simulink model "HW7_2"  (R2021a)
settings: Solver=VariableStepAuto  StartTime=0.0  StopTime=80  RelTol=1e-3
undefined symbols (not defined in the file): f, f_64
libraries: hdlBasic x991, xbsIndex_r4 x1, simulink x1
(part 6 of 6)

== system HW7_2/FIR_64/FIR-transposed1 ==
  In1 : Inport
  In2 : Inport  Port=2
  AddSub{7..11} (5 alike) : hdlBasic/AddSub  mode=Addition  use_carryin=off  use_carryout=off  en=off  latency=0  precision=User Defined  arith_type="Signed  (2's comp)"  n_bits=16  bin_pt=8  quantization=Truncate  overflow=Saturate  use_behavioral_HDL=off  hw_selection=Fabric  pipelined=off  XmcBlockStatus=1  maskContainerNames=tabcontainer1  block_type=addsub  block_config=sysgen:Addsub_config
  AddSub12 : hdlBasic/AddSub  mode=Addition  use_carryin=off  use_carryout=off  en=off  latency=0  precision=User Defined  arith_type=Unsigned  n_bits=16  bin_pt=8  quantization=Truncate  overflow=Saturate  use_behavioral_HDL=off  hw_selection=Fabric  pipelined=off  XmcBlockStatus=1  maskContainerNames=tabcontainer1  block_type=addsub  block_config=sysgen:Addsub_config
  CMult10 : hdlBasic/CMult  const=f(5)  gui_display_data_type=Fixed-point  const_n_bits=8  const_bin_pt=4  float_type=Single  exp_bits=8  fraction_bits=24  en=off  latency=0  precision=User Defined  arith_type="Signed  (2's comp)"  n_bits=16  bin_pt=8  quantization=Truncate  overflow=Saturate  use_behavioral_HDL=off  mem_type=Block RAM  pipeline=off  XmcBlockStatus=1  maskContainerNames=tabcontainer1  block_type=cmult  block_config=sysgen:CMult_config
      settings: infoedit=[]
  CMult11 : hdlBasic/CMult  const=f(6)  gui_display_data_type=Fixed-point  const_n_bits=8  const_bin_pt=4  float_type=Single  exp_bits=8  fraction_bits=24  en=off  latency=0  precision=User Defined  arith_type="Signed  (2's comp)"  n_bits=16  bin_pt=8  quantization=Truncate  overflow=Saturate  use_behavioral_HDL=off  mem_type=Block RAM  pipeline=off  XmcBlockStatus=1  maskContainerNames=tabcontainer1  block_type=cmult  block_config=sysgen:CMult_config
      settings: infoedit=[]
  CMult12 : hdlBasic/CMult  const=f(4)  gui_display_data_type=Fixed-point  const_n_bits=8  const_bin_pt=4  float_type=Single  exp_bits=8  fraction_bits=24  en=off  latency=0  precision=User Defined  arith_type="Signed  (2's comp)"  n_bits=16  bin_pt=8  quantization=Truncate  overflow=Saturate  use_behavioral_HDL=off  mem_type=Block RAM  pipeline=off  XmcBlockStatus=1  maskContainerNames=tabcontainer1  block_type=cmult  block_config=sysgen:CMult_config
      settings: infoedit=[]
  CMult13 : hdlBasic/CMult  const=f(3)  gui_display_data_type=Fixed-point  const_n_bits=8  const_bin_pt=4  float_type=Single  exp_bits=8  fraction_bits=24  en=off  latency=0  precision=User Defined  arith_type="Signed  (2's comp)"  n_bits=16  bin_pt=8  quantization=Truncate  overflow=Saturate  use_behavioral_HDL=off  mem_type=Block RAM  pipeline=off  XmcBlockStatus=1  maskContainerNames=tabcontainer1  block_type=cmult  block_config=sysgen:CMult_config
      settings: infoedit=[]
  CMult14 : hdlBasic/CMult  const=f(2)  gui_display_data_type=Fixed-point  const_n_bits=8  const_bin_pt=4  float_type=Single  exp_bits=8  fraction_bits=24  en=off  latency=0  precision=User Defined  arith_type="Signed  (2's comp)"  n_bits=16  bin_pt=8  quantization=Truncate  overflow=Saturate  use_behavioral_HDL=off  mem_type=Block RAM  pipeline=off  XmcBlockStatus=1  maskContainerNames=tabcontainer1  block_type=cmult  block_config=sysgen:CMult_config
      settings: infoedit=[]
  CMult15 : hdlBasic/CMult  const=f(1)  gui_display_data_type=Fixed-point  const_n_bits=8  const_bin_pt=4  float_type=Single  exp_bits=8  fraction_bits=24  en=off  latency=0  precision=User Defined  arith_type="Signed  (2's comp)"  n_bits=16  bin_pt=8  quantization=Truncate  overflow=Saturate  use_behavioral_HDL=off  mem_type=Block RAM  pipeline=off  XmcBlockStatus=1  maskContainerNames=tabcontainer1  block_type=cmult  block_config=sysgen:CMult_config
      settings: infoedit=[]
  CMult8 : hdlBasic/CMult  const=f(8)  gui_display_data_type=Fixed-point  const_n_bits=8  const_bin_pt=4  float_type=Single  exp_bits=8  fraction_bits=24  en=off  latency=0  precision=User Defined  arith_type="Signed  (2's comp)"  n_bits=16  bin_pt=8  quantization=Truncate  overflow=Saturate  use_behavioral_HDL=off  mem_type=Block RAM  pipeline=off  XmcBlockStatus=1  maskContainerNames=tabcontainer1  block_type=cmult  block_config=sysgen:CMult_config
      settings: infoedit=[]
  CMult9 : hdlBasic/CMult  const=f(7)  gui_display_data_type=Fixed-point  const_n_bits=8  const_bin_pt=4  float_type=Single  exp_bits=8  fraction_bits=24  en=off  latency=0  precision=User Defined  arith_type="Signed  (2's comp)"  n_bits=16  bin_pt=8  quantization=Truncate  overflow=Saturate  use_behavioral_HDL=off  mem_type=Block RAM  pipeline=off  XmcBlockStatus=1  maskContainerNames=tabcontainer1  block_type=cmult  block_config=sysgen:CMult_config
      settings: infoedit=[]
  Delay{1,7..13} (8 alike) : hdlBasic/Delay  rst=off  en=off  latency=1  reg_retiming=off  XmcBlockStatus=1  maskContainerNames=group1  block_type=delay  block_config=sysgen:Delay_config
  Transposed : hdlBasic/AddSub  mode=Addition  use_carryin=off  use_carryout=off  en=off  latency=0  precision=User Defined  arith_type="Signed  (2's comp)"  n_bits=16  bin_pt=8  quantization=Truncate  overflow=Saturate  use_behavioral_HDL=off  hw_selection=Fabric  pipelined=off  XmcBlockStatus=1  maskContainerNames=tabcontainer1  block_type=addsub  block_config=sysgen:Addsub_config
  Transposed1 : hdlBasic/AddSub  mode=Addition  use_carryin=off  use_carryout=off  en=off  latency=0  precision=User Defined  arith_type="Signed  (2's comp)"  n_bits=16  bin_pt=8  quantization=Truncate  overflow=Saturate  use_behavioral_HDL=off  hw_selection=Fabric  pipelined=off  XmcBlockStatus=1  maskContainerNames=tabcontainer1  block_type=addsub  block_config=sysgen:Addsub_config
  Out1 : Outport
  Out2 : Outport  Port=2
  wires:
  Delay12/1 -> AddSub12/2
  CMult10/1 -> AddSub9/1
  AddSub12/1 -> Delay13/1
  Delay9/1 -> AddSub9/2
  CMult9/1 -> AddSub7/1
  AddSub11/1 -> Delay12/1
  Delay10/1 -> AddSub10/2
  AddSub8/1 -> Delay9/1
  CMult11/1 -> AddSub8/1
  Delay8/1 -> AddSub8/2
  CMult12/1 -> AddSub10/1
  Delay11/1 -> AddSub11/2
  AddSub10/1 -> Delay11/1
  CMult14/1 -> AddSub12/1
  CMult15/1 -> Transposed/1
  Delay7/1 -> AddSub7/2
  CMult13/1 -> AddSub11/1
  Delay13/1 -> Transposed/2
  AddSub7/1 -> Delay8/1
  AddSub9/1 -> Delay10/1
  In1/1 -> CMult8/1, Out1/1, CMult15/1, CMult14/1, CMult13/1, CMult12/1, CMult10/1, CMult11/1, CMult9/1
  Transposed/1 -> Out2/1
  Transposed1/1 -> Delay7/1
  CMult8/1 -> Transposed1/1
  Delay1/1 -> Transposed1/2
  In2/1 -> Delay1/1

== system HW7_2/FIR_64/FIR-transposed2 ==
  In1 : Inport
  In2 : Inport  Port=2
  AddSub{7..11} (5 alike) : hdlBasic/AddSub  mode=Addition  use_carryin=off  use_carryout=off  en=off  latency=0  precision=User Defined  arith_type="Signed  (2's comp)"  n_bits=16  bin_pt=8  quantization=Truncate  overflow=Saturate  use_behavioral_HDL=off  hw_selection=Fabric  pipelined=off  XmcBlockStatus=1  maskContainerNames=tabcontainer1  block_type=addsub  block_config=sysgen:Addsub_config
  AddSub12 : hdlBasic/AddSub  mode=Addition  use_carryin=off  use_carryout=off  en=off  latency=0  precision=User Defined  arith_type=Unsigned  n_bits=16  bin_pt=8  quantization=Truncate  overflow=Saturate  use_behavioral_HDL=off  hw_selection=Fabric  pipelined=off  XmcBlockStatus=1  maskContainerNames=tabcontainer1  block_type=addsub  block_config=sysgen:Addsub_config
  CMult10 : hdlBasic/CMult  const=f(5)  gui_display_data_type=Fixed-point  const_n_bits=8  const_bin_pt=4  float_type=Single  exp_bits=8  fraction_bits=24  en=off  latency=0  precision=User Defined  arith_type="Signed  (2's comp)"  n_bits=16  bin_pt=8  quantization=Truncate  overflow=Saturate  use_behavioral_HDL=off  mem_type=Block RAM  pipeline=off  XmcBlockStatus=1  maskContainerNames=tabcontainer1  block_type=cmult  block_config=sysgen:CMult_config
      settings: infoedit=[]
  CMult11 : hdlBasic/CMult  const=f(6)  gui_display_data_type=Fixed-point  const_n_bits=8  const_bin_pt=4  float_type=Single  exp_bits=8  fraction_bits=24  en=off  latency=0  precision=User Defined  arith_type="Signed  (2's comp)"  n_bits=16  bin_pt=8  quantization=Truncate  overflow=Saturate  use_behavioral_HDL=off  mem_type=Block RAM  pipeline=off  XmcBlockStatus=1  maskContainerNames=tabcontainer1  block_type=cmult  block_config=sysgen:CMult_config
      settings: infoedit=[]
  CMult12 : hdlBasic/CMult  const=f(4)  gui_display_data_type=Fixed-point  const_n_bits=8  const_bin_pt=4  float_type=Single  exp_bits=8  fraction_bits=24  en=off  latency=0  precision=User Defined  arith_type="Signed  (2's comp)"  n_bits=16  bin_pt=8  quantization=Truncate  overflow=Saturate  use_behavioral_HDL=off  mem_type=Block RAM  pipeline=off  XmcBlockStatus=1  maskContainerNames=tabcontainer1  block_type=cmult  block_config=sysgen:CMult_config
      settings: infoedit=[]
  CMult13 : hdlBasic/CMult  const=f(3)  gui_display_data_type=Fixed-point  const_n_bits=8  const_bin_pt=4  float_type=Single  exp_bits=8  fraction_bits=24  en=off  latency=0  precision=User Defined  arith_type="Signed  (2's comp)"  n_bits=16  bin_pt=8  quantization=Truncate  overflow=Saturate  use_behavioral_HDL=off  mem_type=Block RAM  pipeline=off  XmcBlockStatus=1  maskContainerNames=tabcontainer1  block_type=cmult  block_config=sysgen:CMult_config
      settings: infoedit=[]
  CMult14 : hdlBasic/CMult  const=f(2)  gui_display_data_type=Fixed-point  const_n_bits=8  const_bin_pt=4  float_type=Single  exp_bits=8  fraction_bits=24  en=off  latency=0  precision=User Defined  arith_type="Signed  (2's comp)"  n_bits=16  bin_pt=8  quantization=Truncate  overflow=Saturate  use_behavioral_HDL=off  mem_type=Block RAM  pipeline=off  XmcBlockStatus=1  maskContainerNames=tabcontainer1  block_type=cmult  block_config=sysgen:CMult_config
      settings: infoedit=[]
  CMult15 : hdlBasic/CMult  const=f(1)  gui_display_data_type=Fixed-point  const_n_bits=8  const_bin_pt=4  float_type=Single  exp_bits=8  fraction_bits=24  en=off  latency=0  precision=User Defined  arith_type="Signed  (2's comp)"  n_bits=16  bin_pt=8  quantization=Truncate  overflow=Saturate  use_behavioral_HDL=off  mem_type=Block RAM  pipeline=off  XmcBlockStatus=1  maskContainerNames=tabcontainer1  block_type=cmult  block_config=sysgen:CMult_config
      settings: infoedit=[]
  CMult8 : hdlBasic/CMult  const=f(8)  gui_display_data_type=Fixed-point  const_n_bits=8  const_bin_pt=4  float_type=Single  exp_bits=8  fraction_bits=24  en=off  latency=0  precision=User Defined  arith_type="Signed  (2's comp)"  n_bits=16  bin_pt=8  quantization=Truncate  overflow=Saturate  use_behavioral_HDL=off  mem_type=Block RAM  pipeline=off  XmcBlockStatus=1  maskContainerNames=tabcontainer1  block_type=cmult  block_config=sysgen:CMult_config
      settings: infoedit=[]
  CMult9 : hdlBasic/CMult  const=f(7)  gui_display_data_type=Fixed-point  const_n_bits=8  const_bin_pt=4  float_type=Single  exp_bits=8  fraction_bits=24  en=off  latency=0  precision=User Defined  arith_type="Signed  (2's comp)"  n_bits=16  bin_pt=8  quantization=Truncate  overflow=Saturate  use_behavioral_HDL=off  mem_type=Block RAM  pipeline=off  XmcBlockStatus=1  maskContainerNames=tabcontainer1  block_type=cmult  block_config=sysgen:CMult_config
      settings: infoedit=[]
  Delay{1,7..13} (8 alike) : hdlBasic/Delay  rst=off  en=off  latency=1  reg_retiming=off  XmcBlockStatus=1  maskContainerNames=group1  block_type=delay  block_config=sysgen:Delay_config
  Transposed : hdlBasic/AddSub  mode=Addition  use_carryin=off  use_carryout=off  en=off  latency=0  precision=User Defined  arith_type="Signed  (2's comp)"  n_bits=16  bin_pt=8  quantization=Truncate  overflow=Saturate  use_behavioral_HDL=off  hw_selection=Fabric  pipelined=off  XmcBlockStatus=1  maskContainerNames=tabcontainer1  block_type=addsub  block_config=sysgen:Addsub_config
  Transposed1 : hdlBasic/AddSub  mode=Addition  use_carryin=off  use_carryout=off  en=off  latency=0  precision=User Defined  arith_type="Signed  (2's comp)"  n_bits=16  bin_pt=8  quantization=Truncate  overflow=Saturate  use_behavioral_HDL=off  hw_selection=Fabric  pipelined=off  XmcBlockStatus=1  maskContainerNames=tabcontainer1  block_type=addsub  block_config=sysgen:Addsub_config
  Out1 : Outport
  Out2 : Outport  Port=2
  wires:
  Delay12/1 -> AddSub12/2
  CMult10/1 -> AddSub9/1
  AddSub12/1 -> Delay13/1
  Delay9/1 -> AddSub9/2
  CMult9/1 -> AddSub7/1
  AddSub11/1 -> Delay12/1
  Delay10/1 -> AddSub10/2
  AddSub8/1 -> Delay9/1
  CMult11/1 -> AddSub8/1
  Delay8/1 -> AddSub8/2
  CMult12/1 -> AddSub10/1
  Delay11/1 -> AddSub11/2
  AddSub10/1 -> Delay11/1
  CMult14/1 -> AddSub12/1
  CMult15/1 -> Transposed/1
  Delay7/1 -> AddSub7/2
  CMult13/1 -> AddSub11/1
  Delay13/1 -> Transposed/2
  AddSub7/1 -> Delay8/1
  AddSub9/1 -> Delay10/1
  In1/1 -> CMult8/1, Out1/1, CMult15/1, CMult14/1, CMult13/1, CMult12/1, CMult10/1, CMult11/1, CMult9/1
  Transposed/1 -> Out2/1
  Transposed1/1 -> Delay7/1
  CMult8/1 -> Transposed1/1
  Delay1/1 -> Transposed1/2
  In2/1 -> Delay1/1

== system HW7_2/FIR_64/FIR-transposed3 ==
  In1 : Inport
  In2 : Inport  Port=2
  AddSub{7..11} (5 alike) : hdlBasic/AddSub  mode=Addition  use_carryin=off  use_carryout=off  en=off  latency=0  precision=User Defined  arith_type="Signed  (2's comp)"  n_bits=16  bin_pt=8  quantization=Truncate  overflow=Saturate  use_behavioral_HDL=off  hw_selection=Fabric  pipelined=off  XmcBlockStatus=1  maskContainerNames=tabcontainer1  block_type=addsub  block_config=sysgen:Addsub_config
  AddSub12 : hdlBasic/AddSub  mode=Addition  use_carryin=off  use_carryout=off  en=off  latency=0  precision=User Defined  arith_type=Unsigned  n_bits=16  bin_pt=8  quantization=Truncate  overflow=Saturate  use_behavioral_HDL=off  hw_selection=Fabric  pipelined=off  XmcBlockStatus=1  maskContainerNames=tabcontainer1  block_type=addsub  block_config=sysgen:Addsub_config
  CMult10 : hdlBasic/CMult  const=f(5)  gui_display_data_type=Fixed-point  const_n_bits=8  const_bin_pt=4  float_type=Single  exp_bits=8  fraction_bits=24  en=off  latency=0  precision=User Defined  arith_type="Signed  (2's comp)"  n_bits=16  bin_pt=8  quantization=Truncate  overflow=Saturate  use_behavioral_HDL=off  mem_type=Block RAM  pipeline=off  XmcBlockStatus=1  maskContainerNames=tabcontainer1  block_type=cmult  block_config=sysgen:CMult_config
      settings: infoedit=[]
  CMult11 : hdlBasic/CMult  const=f(6)  gui_display_data_type=Fixed-point  const_n_bits=8  const_bin_pt=4  float_type=Single  exp_bits=8  fraction_bits=24  en=off  latency=0  precision=User Defined  arith_type="Signed  (2's comp)"  n_bits=16  bin_pt=8  quantization=Truncate  overflow=Saturate  use_behavioral_HDL=off  mem_type=Block RAM  pipeline=off  XmcBlockStatus=1  maskContainerNames=tabcontainer1  block_type=cmult  block_config=sysgen:CMult_config
      settings: infoedit=[]
  CMult12 : hdlBasic/CMult  const=f(4)  gui_display_data_type=Fixed-point  const_n_bits=8  const_bin_pt=4  float_type=Single  exp_bits=8  fraction_bits=24  en=off  latency=0  precision=User Defined  arith_type="Signed  (2's comp)"  n_bits=16  bin_pt=8  quantization=Truncate  overflow=Saturate  use_behavioral_HDL=off  mem_type=Block RAM  pipeline=off  XmcBlockStatus=1  maskContainerNames=tabcontainer1  block_type=cmult  block_config=sysgen:CMult_config
      settings: infoedit=[]
  CMult13 : hdlBasic/CMult  const=f(3)  gui_display_data_type=Fixed-point  const_n_bits=8  const_bin_pt=4  float_type=Single  exp_bits=8  fraction_bits=24  en=off  latency=0  precision=User Defined  arith_type="Signed  (2's comp)"  n_bits=16  bin_pt=8  quantization=Truncate  overflow=Saturate  use_behavioral_HDL=off  mem_type=Block RAM  pipeline=off  XmcBlockStatus=1  maskContainerNames=tabcontainer1  block_type=cmult  block_config=sysgen:CMult_config
      settings: infoedit=[]
  CMult14 : hdlBasic/CMult  const=f(2)  gui_display_data_type=Fixed-point  const_n_bits=8  const_bin_pt=4  float_type=Single  exp_bits=8  fraction_bits=24  en=off  latency=0  precision=User Defined  arith_type="Signed  (2's comp)"  n_bits=16  bin_pt=8  quantization=Truncate  overflow=Saturate  use_behavioral_HDL=off  mem_type=Block RAM  pipeline=off  XmcBlockStatus=1  maskContainerNames=tabcontainer1  block_type=cmult  block_config=sysgen:CMult_config
      settings: infoedit=[]
  CMult15 : hdlBasic/CMult  const=f(1)  gui_display_data_type=Fixed-point  const_n_bits=8  const_bin_pt=4  float_type=Single  exp_bits=8  fraction_bits=24  en=off  latency=0  precision=User Defined  arith_type="Signed  (2's comp)"  n_bits=16  bin_pt=8  quantization=Truncate  overflow=Saturate  use_behavioral_HDL=off  mem_type=Block RAM  pipeline=off  XmcBlockStatus=1  maskContainerNames=tabcontainer1  block_type=cmult  block_config=sysgen:CMult_config
      settings: infoedit=[]
  CMult8 : hdlBasic/CMult  const=f(8)  gui_display_data_type=Fixed-point  const_n_bits=8  const_bin_pt=4  float_type=Single  exp_bits=8  fraction_bits=24  en=off  latency=0  precision=User Defined  arith_type="Signed  (2's comp)"  n_bits=16  bin_pt=8  quantization=Truncate  overflow=Saturate  use_behavioral_HDL=off  mem_type=Block RAM  pipeline=off  XmcBlockStatus=1  maskContainerNames=tabcontainer1  block_type=cmult  block_config=sysgen:CMult_config
      settings: infoedit=[]
  CMult9 : hdlBasic/CMult  const=f(7)  gui_display_data_type=Fixed-point  const_n_bits=8  const_bin_pt=4  float_type=Single  exp_bits=8  fraction_bits=24  en=off  latency=0  precision=User Defined  arith_type="Signed  (2's comp)"  n_bits=16  bin_pt=8  quantization=Truncate  overflow=Saturate  use_behavioral_HDL=off  mem_type=Block RAM  pipeline=off  XmcBlockStatus=1  maskContainerNames=tabcontainer1  block_type=cmult  block_config=sysgen:CMult_config
      settings: infoedit=[]
  Delay{1,7..13} (8 alike) : hdlBasic/Delay  rst=off  en=off  latency=1  reg_retiming=off  XmcBlockStatus=1  maskContainerNames=group1  block_type=delay  block_config=sysgen:Delay_config
  Transposed : hdlBasic/AddSub  mode=Addition  use_carryin=off  use_carryout=off  en=off  latency=0  precision=User Defined  arith_type="Signed  (2's comp)"  n_bits=16  bin_pt=8  quantization=Truncate  overflow=Saturate  use_behavioral_HDL=off  hw_selection=Fabric  pipelined=off  XmcBlockStatus=1  maskContainerNames=tabcontainer1  block_type=addsub  block_config=sysgen:Addsub_config
  Transposed1 : hdlBasic/AddSub  mode=Addition  use_carryin=off  use_carryout=off  en=off  latency=0  precision=User Defined  arith_type="Signed  (2's comp)"  n_bits=16  bin_pt=8  quantization=Truncate  overflow=Saturate  use_behavioral_HDL=off  hw_selection=Fabric  pipelined=off  XmcBlockStatus=1  maskContainerNames=tabcontainer1  block_type=addsub  block_config=sysgen:Addsub_config
  Out1 : Outport
  Out2 : Outport  Port=2
  wires:
  Delay12/1 -> AddSub12/2
  CMult10/1 -> AddSub9/1
  AddSub12/1 -> Delay13/1
  Delay9/1 -> AddSub9/2
  CMult9/1 -> AddSub7/1
  AddSub11/1 -> Delay12/1
  Delay10/1 -> AddSub10/2
  AddSub8/1 -> Delay9/1
  CMult11/1 -> AddSub8/1
  Delay8/1 -> AddSub8/2
  CMult12/1 -> AddSub10/1
  Delay11/1 -> AddSub11/2
  AddSub10/1 -> Delay11/1
  CMult14/1 -> AddSub12/1
  CMult15/1 -> Transposed/1
  Delay7/1 -> AddSub7/2
  CMult13/1 -> AddSub11/1
  Delay13/1 -> Transposed/2
  AddSub7/1 -> Delay8/1
  AddSub9/1 -> Delay10/1
  In1/1 -> CMult8/1, Out1/1, CMult15/1, CMult14/1, CMult13/1, CMult12/1, CMult10/1, CMult11/1, CMult9/1
  Transposed/1 -> Out2/1
  Transposed1/1 -> Delay7/1
  CMult8/1 -> Transposed1/1
  Delay1/1 -> Transposed1/2
  In2/1 -> Delay1/1

== system HW7_2/FIR_64/FIR-transposed4 ==
  In1 : Inport
  In2 : Inport  Port=2
  AddSub{7..11} (5 alike) : hdlBasic/AddSub  mode=Addition  use_carryin=off  use_carryout=off  en=off  latency=0  precision=User Defined  arith_type="Signed  (2's comp)"  n_bits=16  bin_pt=8  quantization=Truncate  overflow=Saturate  use_behavioral_HDL=off  hw_selection=Fabric  pipelined=off  XmcBlockStatus=1  maskContainerNames=tabcontainer1  block_type=addsub  block_config=sysgen:Addsub_config
  AddSub12 : hdlBasic/AddSub  mode=Addition  use_carryin=off  use_carryout=off  en=off  latency=0  precision=User Defined  arith_type=Unsigned  n_bits=16  bin_pt=8  quantization=Truncate  overflow=Saturate  use_behavioral_HDL=off  hw_selection=Fabric  pipelined=off  XmcBlockStatus=1  maskContainerNames=tabcontainer1  block_type=addsub  block_config=sysgen:Addsub_config
  CMult10 : hdlBasic/CMult  const=f(5)  gui_display_data_type=Fixed-point  const_n_bits=8  const_bin_pt=4  float_type=Single  exp_bits=8  fraction_bits=24  en=off  latency=0  precision=User Defined  arith_type="Signed  (2's comp)"  n_bits=16  bin_pt=8  quantization=Truncate  overflow=Saturate  use_behavioral_HDL=off  mem_type=Block RAM  pipeline=off  XmcBlockStatus=1  maskContainerNames=tabcontainer1  block_type=cmult  block_config=sysgen:CMult_config
      settings: infoedit=[]
  CMult11 : hdlBasic/CMult  const=f(6)  gui_display_data_type=Fixed-point  const_n_bits=8  const_bin_pt=4  float_type=Single  exp_bits=8  fraction_bits=24  en=off  latency=0  precision=User Defined  arith_type="Signed  (2's comp)"  n_bits=16  bin_pt=8  quantization=Truncate  overflow=Saturate  use_behavioral_HDL=off  mem_type=Block RAM  pipeline=off  XmcBlockStatus=1  maskContainerNames=tabcontainer1  block_type=cmult  block_config=sysgen:CMult_config
      settings: infoedit=[]
  CMult12 : hdlBasic/CMult  const=f(4)  gui_display_data_type=Fixed-point  const_n_bits=8  const_bin_pt=4  float_type=Single  exp_bits=8  fraction_bits=24  en=off  latency=0  precision=User Defined  arith_type="Signed  (2's comp)"  n_bits=16  bin_pt=8  quantization=Truncate  overflow=Saturate  use_behavioral_HDL=off  mem_type=Block RAM  pipeline=off  XmcBlockStatus=1  maskContainerNames=tabcontainer1  block_type=cmult  block_config=sysgen:CMult_config
      settings: infoedit=[]
  CMult13 : hdlBasic/CMult  const=f(3)  gui_display_data_type=Fixed-point  const_n_bits=8  const_bin_pt=4  float_type=Single  exp_bits=8  fraction_bits=24  en=off  latency=0  precision=User Defined  arith_type="Signed  (2's comp)"  n_bits=16  bin_pt=8  quantization=Truncate  overflow=Saturate  use_behavioral_HDL=off  mem_type=Block RAM  pipeline=off  XmcBlockStatus=1  maskContainerNames=tabcontainer1  block_type=cmult  block_config=sysgen:CMult_config
      settings: infoedit=[]
  CMult14 : hdlBasic/CMult  const=f(2)  gui_display_data_type=Fixed-point  const_n_bits=8  const_bin_pt=4  float_type=Single  exp_bits=8  fraction_bits=24  en=off  latency=0  precision=User Defined  arith_type="Signed  (2's comp)"  n_bits=16  bin_pt=8  quantization=Truncate  overflow=Saturate  use_behavioral_HDL=off  mem_type=Block RAM  pipeline=off  XmcBlockStatus=1  maskContainerNames=tabcontainer1  block_type=cmult  block_config=sysgen:CMult_config
      settings: infoedit=[]
  CMult15 : hdlBasic/CMult  const=f(1)  gui_display_data_type=Fixed-point  const_n_bits=8  const_bin_pt=4  float_type=Single  exp_bits=8  fraction_bits=24  en=off  latency=0  precision=User Defined  arith_type="Signed  (2's comp)"  n_bits=16  bin_pt=8  quantization=Truncate  overflow=Saturate  use_behavioral_HDL=off  mem_type=Block RAM  pipeline=off  XmcBlockStatus=1  maskContainerNames=tabcontainer1  block_type=cmult  block_config=sysgen:CMult_config
      settings: infoedit=[]
  CMult8 : hdlBasic/CMult  const=f(8)  gui_display_data_type=Fixed-point  const_n_bits=8  const_bin_pt=4  float_type=Single  exp_bits=8  fraction_bits=24  en=off  latency=0  precision=User Defined  arith_type="Signed  (2's comp)"  n_bits=16  bin_pt=8  quantization=Truncate  overflow=Saturate  use_behavioral_HDL=off  mem_type=Block RAM  pipeline=off  XmcBlockStatus=1  maskContainerNames=tabcontainer1  block_type=cmult  block_config=sysgen:CMult_config
      settings: infoedit=[]
  CMult9 : hdlBasic/CMult  const=f(7)  gui_display_data_type=Fixed-point  const_n_bits=8  const_bin_pt=4  float_type=Single  exp_bits=8  fraction_bits=24  en=off  latency=0  precision=User Defined  arith_type="Signed  (2's comp)"  n_bits=16  bin_pt=8  quantization=Truncate  overflow=Saturate  use_behavioral_HDL=off  mem_type=Block RAM  pipeline=off  XmcBlockStatus=1  maskContainerNames=tabcontainer1  block_type=cmult  block_config=sysgen:CMult_config
      settings: infoedit=[]
  Delay{1,7..13} (8 alike) : hdlBasic/Delay  rst=off  en=off  latency=1  reg_retiming=off  XmcBlockStatus=1  maskContainerNames=group1  block_type=delay  block_config=sysgen:Delay_config
  Transposed : hdlBasic/AddSub  mode=Addition  use_carryin=off  use_carryout=off  en=off  latency=0  precision=User Defined  arith_type="Signed  (2's comp)"  n_bits=16  bin_pt=8  quantization=Truncate  overflow=Saturate  use_behavioral_HDL=off  hw_selection=Fabric  pipelined=off  XmcBlockStatus=1  maskContainerNames=tabcontainer1  block_type=addsub  block_config=sysgen:Addsub_config
  Transposed1 : hdlBasic/AddSub  mode=Addition  use_carryin=off  use_carryout=off  en=off  latency=0  precision=User Defined  arith_type="Signed  (2's comp)"  n_bits=16  bin_pt=8  quantization=Truncate  overflow=Saturate  use_behavioral_HDL=off  hw_selection=Fabric  pipelined=off  XmcBlockStatus=1  maskContainerNames=tabcontainer1  block_type=addsub  block_config=sysgen:Addsub_config
  Out1 : Outport
  Out2 : Outport  Port=2
  wires:
  Delay12/1 -> AddSub12/2
  CMult10/1 -> AddSub9/1
  AddSub12/1 -> Delay13/1
  Delay9/1 -> AddSub9/2
  CMult9/1 -> AddSub7/1
  AddSub11/1 -> Delay12/1
  Delay10/1 -> AddSub10/2
  AddSub8/1 -> Delay9/1
  CMult11/1 -> AddSub8/1
  Delay8/1 -> AddSub8/2
  CMult12/1 -> AddSub10/1
  Delay11/1 -> AddSub11/2
  AddSub10/1 -> Delay11/1
  CMult14/1 -> AddSub12/1
  CMult15/1 -> Transposed/1
  Delay7/1 -> AddSub7/2
  CMult13/1 -> AddSub11/1
  Delay13/1 -> Transposed/2
  AddSub7/1 -> Delay8/1
  AddSub9/1 -> Delay10/1
  In1/1 -> CMult8/1, Out1/1, CMult15/1, CMult14/1, CMult13/1, CMult12/1, CMult10/1, CMult11/1, CMult9/1
  Transposed/1 -> Out2/1
  Transposed1/1 -> Delay7/1
  CMult8/1 -> Transposed1/1
  Delay1/1 -> Transposed1/2
  In2/1 -> Delay1/1

== system HW7_2/FIR_64/FIR-transposed5 ==
  In1 : Inport
  In2 : Inport  Port=2
  AddSub{7..11} (5 alike) : hdlBasic/AddSub  mode=Addition  use_carryin=off  use_carryout=off  en=off  latency=0  precision=User Defined  arith_type="Signed  (2's comp)"  n_bits=16  bin_pt=8  quantization=Truncate  overflow=Saturate  use_behavioral_HDL=off  hw_selection=Fabric  pipelined=off  XmcBlockStatus=1  maskContainerNames=tabcontainer1  block_type=addsub  block_config=sysgen:Addsub_config
  AddSub12 : hdlBasic/AddSub  mode=Addition  use_carryin=off  use_carryout=off  en=off  latency=0  precision=User Defined  arith_type=Unsigned  n_bits=16  bin_pt=8  quantization=Truncate  overflow=Saturate  use_behavioral_HDL=off  hw_selection=Fabric  pipelined=off  XmcBlockStatus=1  maskContainerNames=tabcontainer1  block_type=addsub  block_config=sysgen:Addsub_config
  CMult10 : hdlBasic/CMult  const=f(5)  gui_display_data_type=Fixed-point  const_n_bits=8  const_bin_pt=4  float_type=Single  exp_bits=8  fraction_bits=24  en=off  latency=0  precision=User Defined  arith_type="Signed  (2's comp)"  n_bits=16  bin_pt=8  quantization=Truncate  overflow=Saturate  use_behavioral_HDL=off  mem_type=Block RAM  pipeline=off  XmcBlockStatus=1  maskContainerNames=tabcontainer1  block_type=cmult  block_config=sysgen:CMult_config
      settings: infoedit=[]
  CMult11 : hdlBasic/CMult  const=f(6)  gui_display_data_type=Fixed-point  const_n_bits=8  const_bin_pt=4  float_type=Single  exp_bits=8  fraction_bits=24  en=off  latency=0  precision=User Defined  arith_type="Signed  (2's comp)"  n_bits=16  bin_pt=8  quantization=Truncate  overflow=Saturate  use_behavioral_HDL=off  mem_type=Block RAM  pipeline=off  XmcBlockStatus=1  maskContainerNames=tabcontainer1  block_type=cmult  block_config=sysgen:CMult_config
      settings: infoedit=[]
  CMult12 : hdlBasic/CMult  const=f(4)  gui_display_data_type=Fixed-point  const_n_bits=8  const_bin_pt=4  float_type=Single  exp_bits=8  fraction_bits=24  en=off  latency=0  precision=User Defined  arith_type="Signed  (2's comp)"  n_bits=16  bin_pt=8  quantization=Truncate  overflow=Saturate  use_behavioral_HDL=off  mem_type=Block RAM  pipeline=off  XmcBlockStatus=1  maskContainerNames=tabcontainer1  block_type=cmult  block_config=sysgen:CMult_config
      settings: infoedit=[]
  CMult13 : hdlBasic/CMult  const=f(3)  gui_display_data_type=Fixed-point  const_n_bits=8  const_bin_pt=4  float_type=Single  exp_bits=8  fraction_bits=24  en=off  latency=0  precision=User Defined  arith_type="Signed  (2's comp)"  n_bits=16  bin_pt=8  quantization=Truncate  overflow=Saturate  use_behavioral_HDL=off  mem_type=Block RAM  pipeline=off  XmcBlockStatus=1  maskContainerNames=tabcontainer1  block_type=cmult  block_config=sysgen:CMult_config
      settings: infoedit=[]
  CMult14 : hdlBasic/CMult  const=f(2)  gui_display_data_type=Fixed-point  const_n_bits=8  const_bin_pt=4  float_type=Single  exp_bits=8  fraction_bits=24  en=off  latency=0  precision=User Defined  arith_type="Signed  (2's comp)"  n_bits=16  bin_pt=8  quantization=Truncate  overflow=Saturate  use_behavioral_HDL=off  mem_type=Block RAM  pipeline=off  XmcBlockStatus=1  maskContainerNames=tabcontainer1  block_type=cmult  block_config=sysgen:CMult_config
      settings: infoedit=[]
  CMult15 : hdlBasic/CMult  const=f(1)  gui_display_data_type=Fixed-point  const_n_bits=8  const_bin_pt=4  float_type=Single  exp_bits=8  fraction_bits=24  en=off  latency=0  precision=User Defined  arith_type="Signed  (2's comp)"  n_bits=16  bin_pt=8  quantization=Truncate  overflow=Saturate  use_behavioral_HDL=off  mem_type=Block RAM  pipeline=off  XmcBlockStatus=1  maskContainerNames=tabcontainer1  block_type=cmult  block_config=sysgen:CMult_config
      settings: infoedit=[]
  CMult8 : hdlBasic/CMult  const=f(8)  gui_display_data_type=Fixed-point  const_n_bits=8  const_bin_pt=4  float_type=Single  exp_bits=8  fraction_bits=24  en=off  latency=0  precision=User Defined  arith_type="Signed  (2's comp)"  n_bits=16  bin_pt=8  quantization=Truncate  overflow=Saturate  use_behavioral_HDL=off  mem_type=Block RAM  pipeline=off  XmcBlockStatus=1  maskContainerNames=tabcontainer1  block_type=cmult  block_config=sysgen:CMult_config
      settings: infoedit=[]
  CMult9 : hdlBasic/CMult  const=f(7)  gui_display_data_type=Fixed-point  const_n_bits=8  const_bin_pt=4  float_type=Single  exp_bits=8  fraction_bits=24  en=off  latency=0  precision=User Defined  arith_type="Signed  (2's comp)"  n_bits=16  bin_pt=8  quantization=Truncate  overflow=Saturate  use_behavioral_HDL=off  mem_type=Block RAM  pipeline=off  XmcBlockStatus=1  maskContainerNames=tabcontainer1  block_type=cmult  block_config=sysgen:CMult_config
      settings: infoedit=[]
  Delay{1,7..13} (8 alike) : hdlBasic/Delay  rst=off  en=off  latency=1  reg_retiming=off  XmcBlockStatus=1  maskContainerNames=group1  block_type=delay  block_config=sysgen:Delay_config
  Transposed : hdlBasic/AddSub  mode=Addition  use_carryin=off  use_carryout=off  en=off  latency=0  precision=User Defined  arith_type="Signed  (2's comp)"  n_bits=16  bin_pt=8  quantization=Truncate  overflow=Saturate  use_behavioral_HDL=off  hw_selection=Fabric  pipelined=off  XmcBlockStatus=1  maskContainerNames=tabcontainer1  block_type=addsub  block_config=sysgen:Addsub_config
  Transposed1 : hdlBasic/AddSub  mode=Addition  use_carryin=off  use_carryout=off  en=off  latency=0  precision=User Defined  arith_type="Signed  (2's comp)"  n_bits=16  bin_pt=8  quantization=Truncate  overflow=Saturate  use_behavioral_HDL=off  hw_selection=Fabric  pipelined=off  XmcBlockStatus=1  maskContainerNames=tabcontainer1  block_type=addsub  block_config=sysgen:Addsub_config
  Out1 : Outport
  Out2 : Outport  Port=2
  wires:
  Delay12/1 -> AddSub12/2
  CMult10/1 -> AddSub9/1
  AddSub12/1 -> Delay13/1
  Delay9/1 -> AddSub9/2
  CMult9/1 -> AddSub7/1
  AddSub11/1 -> Delay12/1
  Delay10/1 -> AddSub10/2
  AddSub8/1 -> Delay9/1
  CMult11/1 -> AddSub8/1
  Delay8/1 -> AddSub8/2
  CMult12/1 -> AddSub10/1
  Delay11/1 -> AddSub11/2
  AddSub10/1 -> Delay11/1
  CMult14/1 -> AddSub12/1
  CMult15/1 -> Transposed/1
  Delay7/1 -> AddSub7/2
  CMult13/1 -> AddSub11/1
  Delay13/1 -> Transposed/2
  AddSub7/1 -> Delay8/1
  AddSub9/1 -> Delay10/1
  In1/1 -> CMult8/1, Out1/1, CMult15/1, CMult14/1, CMult13/1, CMult12/1, CMult10/1, CMult11/1, CMult9/1
  Transposed/1 -> Out2/1
  Transposed1/1 -> Delay7/1
  CMult8/1 -> Transposed1/1
  Delay1/1 -> Transposed1/2
  In2/1 -> Delay1/1

== system HW7_2/FIR_64/FIR-transposed6 ==
  In1 : Inport
  In2 : Inport  Port=2
  AddSub{7..11} (5 alike) : hdlBasic/AddSub  mode=Addition  use_carryin=off  use_carryout=off  en=off  latency=0  precision=User Defined  arith_type="Signed  (2's comp)"  n_bits=16  bin_pt=8  quantization=Truncate  overflow=Saturate  use_behavioral_HDL=off  hw_selection=Fabric  pipelined=off  XmcBlockStatus=1  maskContainerNames=tabcontainer1  block_type=addsub  block_config=sysgen:Addsub_config
  AddSub12 : hdlBasic/AddSub  mode=Addition  use_carryin=off  use_carryout=off  en=off  latency=0  precision=User Defined  arith_type=Unsigned  n_bits=16  bin_pt=8  quantization=Truncate  overflow=Saturate  use_behavioral_HDL=off  hw_selection=Fabric  pipelined=off  XmcBlockStatus=1  maskContainerNames=tabcontainer1  block_type=addsub  block_config=sysgen:Addsub_config
  CMult10 : hdlBasic/CMult  const=f(5)  gui_display_data_type=Fixed-point  const_n_bits=8  const_bin_pt=4  float_type=Single  exp_bits=8  fraction_bits=24  en=off  latency=0  precision=User Defined  arith_type="Signed  (2's comp)"  n_bits=16  bin_pt=8  quantization=Truncate  overflow=Saturate  use_behavioral_HDL=off  mem_type=Block RAM  pipeline=off  XmcBlockStatus=1  maskContainerNames=tabcontainer1  block_type=cmult  block_config=sysgen:CMult_config
      settings: infoedit=[]
  CMult11 : hdlBasic/CMult  const=f(6)  gui_display_data_type=Fixed-point  const_n_bits=8  const_bin_pt=4  float_type=Single  exp_bits=8  fraction_bits=24  en=off  latency=0  precision=User Defined  arith_type="Signed  (2's comp)"  n_bits=16  bin_pt=8  quantization=Truncate  overflow=Saturate  use_behavioral_HDL=off  mem_type=Block RAM  pipeline=off  XmcBlockStatus=1  maskContainerNames=tabcontainer1  block_type=cmult  block_config=sysgen:CMult_config
      settings: infoedit=[]
  CMult12 : hdlBasic/CMult  const=f(4)  gui_display_data_type=Fixed-point  const_n_bits=8  const_bin_pt=4  float_type=Single  exp_bits=8  fraction_bits=24  en=off  latency=0  precision=User Defined  arith_type="Signed  (2's comp)"  n_bits=16  bin_pt=8  quantization=Truncate  overflow=Saturate  use_behavioral_HDL=off  mem_type=Block RAM  pipeline=off  XmcBlockStatus=1  maskContainerNames=tabcontainer1  block_type=cmult  block_config=sysgen:CMult_config
      settings: infoedit=[]
  CMult13 : hdlBasic/CMult  const=f(3)  gui_display_data_type=Fixed-point  const_n_bits=8  const_bin_pt=4  float_type=Single  exp_bits=8  fraction_bits=24  en=off  latency=0  precision=User Defined  arith_type="Signed  (2's comp)"  n_bits=16  bin_pt=8  quantization=Truncate  overflow=Saturate  use_behavioral_HDL=off  mem_type=Block RAM  pipeline=off  XmcBlockStatus=1  maskContainerNames=tabcontainer1  block_type=cmult  block_config=sysgen:CMult_config
      settings: infoedit=[]
  CMult14 : hdlBasic/CMult  const=f(2)  gui_display_data_type=Fixed-point  const_n_bits=8  const_bin_pt=4  float_type=Single  exp_bits=8  fraction_bits=24  en=off  latency=0  precision=User Defined  arith_type="Signed  (2's comp)"  n_bits=16  bin_pt=8  quantization=Truncate  overflow=Saturate  use_behavioral_HDL=off  mem_type=Block RAM  pipeline=off  XmcBlockStatus=1  maskContainerNames=tabcontainer1  block_type=cmult  block_config=sysgen:CMult_config
      settings: infoedit=[]
  CMult15 : hdlBasic/CMult  const=f(1)  gui_display_data_type=Fixed-point  const_n_bits=8  const_bin_pt=4  float_type=Single  exp_bits=8  fraction_bits=24  en=off  latency=0  precision=User Defined  arith_type="Signed  (2's comp)"  n_bits=16  bin_pt=8  quantization=Truncate  overflow=Saturate  use_behavioral_HDL=off  mem_type=Block RAM  pipeline=off  XmcBlockStatus=1  maskContainerNames=tabcontainer1  block_type=cmult  block_config=sysgen:CMult_config
      settings: infoedit=[]
  CMult8 : hdlBasic/CMult  const=f(8)  gui_display_data_type=Fixed-point  const_n_bits=8  const_bin_pt=4  float_type=Single  exp_bits=8  fraction_bits=24  en=off  latency=0  precision=User Defined  arith_type="Signed  (2's comp)"  n_bits=16  bin_pt=8  quantization=Truncate  overflow=Saturate  use_behavioral_HDL=off  mem_type=Block RAM  pipeline=off  XmcBlockStatus=1  maskContainerNames=tabcontainer1  block_type=cmult  block_config=sysgen:CMult_config
      settings: infoedit=[]
  CMult9 : hdlBasic/CMult  const=f(7)  gui_display_data_type=Fixed-point  const_n_bits=8  const_bin_pt=4  float_type=Single  exp_bits=8  fraction_bits=24  en=off  latency=0  precision=User Defined  arith_type="Signed  (2's comp)"  n_bits=16  bin_pt=8  quantization=Truncate  overflow=Saturate  use_behavioral_HDL=off  mem_type=Block RAM  pipeline=off  XmcBlockStatus=1  maskContainerNames=tabcontainer1  block_type=cmult  block_config=sysgen:CMult_config
      settings: infoedit=[]
  Delay{1,7..13} (8 alike) : hdlBasic/Delay  rst=off  en=off  latency=1  reg_retiming=off  XmcBlockStatus=1  maskContainerNames=group1  block_type=delay  block_config=sysgen:Delay_config
  Transposed : hdlBasic/AddSub  mode=Addition  use_carryin=off  use_carryout=off  en=off  latency=0  precision=User Defined  arith_type="Signed  (2's comp)"  n_bits=16  bin_pt=8  quantization=Truncate  overflow=Saturate  use_behavioral_HDL=off  hw_selection=Fabric  pipelined=off  XmcBlockStatus=1  maskContainerNames=tabcontainer1  block_type=addsub  block_config=sysgen:Addsub_config
  Transposed1 : hdlBasic/AddSub  mode=Addition  use_carryin=off  use_carryout=off  en=off  latency=0  precision=User Defined  arith_type="Signed  (2's comp)"  n_bits=16  bin_pt=8  quantization=Truncate  overflow=Saturate  use_behavioral_HDL=off  hw_selection=Fabric  pipelined=off  XmcBlockStatus=1  maskContainerNames=tabcontainer1  block_type=addsub  block_config=sysgen:Addsub_config
  Out1 : Outport
  Out2 : Outport  Port=2
  wires:
  Delay12/1 -> AddSub12/2
  CMult10/1 -> AddSub9/1
  AddSub12/1 -> Delay13/1
  Delay9/1 -> AddSub9/2
  CMult9/1 -> AddSub7/1
  AddSub11/1 -> Delay12/1
  Delay10/1 -> AddSub10/2
  AddSub8/1 -> Delay9/1
  CMult11/1 -> AddSub8/1
  Delay8/1 -> AddSub8/2
  CMult12/1 -> AddSub10/1
  Delay11/1 -> AddSub11/2
  AddSub10/1 -> Delay11/1
  CMult14/1 -> AddSub12/1
  CMult15/1 -> Transposed/1
  Delay7/1 -> AddSub7/2
  CMult13/1 -> AddSub11/1
  Delay13/1 -> Transposed/2
  AddSub7/1 -> Delay8/1
  AddSub9/1 -> Delay10/1
  In1/1 -> CMult8/1, Out1/1, CMult15/1, CMult14/1, CMult13/1, CMult12/1, CMult10/1, CMult11/1, CMult9/1
  Transposed/1 -> Out2/1
  Transposed1/1 -> Delay7/1
  CMult8/1 -> Transposed1/1
  Delay1/1 -> Transposed1/2
  In2/1 -> Delay1/1

== system HW7_2/FIR_64/FIR-transposed7 ==
  In1 : Inport
  In2 : Inport  Port=2
  AddSub{7..11} (5 alike) : hdlBasic/AddSub  mode=Addition  use_carryin=off  use_carryout=off  en=off  latency=0  precision=User Defined  arith_type="Signed  (2's comp)"  n_bits=16  bin_pt=8  quantization=Truncate  overflow=Saturate  use_behavioral_HDL=off  hw_selection=Fabric  pipelined=off  XmcBlockStatus=1  maskContainerNames=tabcontainer1  block_type=addsub  block_config=sysgen:Addsub_config
  AddSub12 : hdlBasic/AddSub  mode=Addition  use_carryin=off  use_carryout=off  en=off  latency=0  precision=User Defined  arith_type=Unsigned  n_bits=16  bin_pt=8  quantization=Truncate  overflow=Saturate  use_behavioral_HDL=off  hw_selection=Fabric  pipelined=off  XmcBlockStatus=1  maskContainerNames=tabcontainer1  block_type=addsub  block_config=sysgen:Addsub_config
  CMult10 : hdlBasic/CMult  const=f(5)  gui_display_data_type=Fixed-point  const_n_bits=8  const_bin_pt=4  float_type=Single  exp_bits=8  fraction_bits=24  en=off  latency=0  precision=User Defined  arith_type="Signed  (2's comp)"  n_bits=16  bin_pt=8  quantization=Truncate  overflow=Saturate  use_behavioral_HDL=off  mem_type=Block RAM  pipeline=off  XmcBlockStatus=1  maskContainerNames=tabcontainer1  block_type=cmult  block_config=sysgen:CMult_config
      settings: infoedit=[]
  CMult11 : hdlBasic/CMult  const=f(6)  gui_display_data_type=Fixed-point  const_n_bits=8  const_bin_pt=4  float_type=Single  exp_bits=8  fraction_bits=24  en=off  latency=0  precision=User Defined  arith_type="Signed  (2's comp)"  n_bits=16  bin_pt=8  quantization=Truncate  overflow=Saturate  use_behavioral_HDL=off  mem_type=Block RAM  pipeline=off  XmcBlockStatus=1  maskContainerNames=tabcontainer1  block_type=cmult  block_config=sysgen:CMult_config
      settings: infoedit=[]
  CMult12 : hdlBasic/CMult  const=f(4)  gui_display_data_type=Fixed-point  const_n_bits=8  const_bin_pt=4  float_type=Single  exp_bits=8  fraction_bits=24  en=off  latency=0  precision=User Defined  arith_type="Signed  (2's comp)"  n_bits=16  bin_pt=8  quantization=Truncate  overflow=Saturate  use_behavioral_HDL=off  mem_type=Block RAM  pipeline=off  XmcBlockStatus=1  maskContainerNames=tabcontainer1  block_type=cmult  block_config=sysgen:CMult_config
      settings: infoedit=[]
  CMult13 : hdlBasic/CMult  const=f(3)  gui_display_data_type=Fixed-point  const_n_bits=8  const_bin_pt=4  float_type=Single  exp_bits=8  fraction_bits=24  en=off  latency=0  precision=User Defined  arith_type="Signed  (2's comp)"  n_bits=16  bin_pt=8  quantization=Truncate  overflow=Saturate  use_behavioral_HDL=off  mem_type=Block RAM  pipeline=off  XmcBlockStatus=1  maskContainerNames=tabcontainer1  block_type=cmult  block_config=sysgen:CMult_config
      settings: infoedit=[]
  CMult14 : hdlBasic/CMult  const=f(2)  gui_display_data_type=Fixed-point  const_n_bits=8  const_bin_pt=4  float_type=Single  exp_bits=8  fraction_bits=24  en=off  latency=0  precision=User Defined  arith_type="Signed  (2's comp)"  n_bits=16  bin_pt=8  quantization=Truncate  overflow=Saturate  use_behavioral_HDL=off  mem_type=Block RAM  pipeline=off  XmcBlockStatus=1  maskContainerNames=tabcontainer1  block_type=cmult  block_config=sysgen:CMult_config
      settings: infoedit=[]
  CMult15 : hdlBasic/CMult  const=f(1)  gui_display_data_type=Fixed-point  const_n_bits=8  const_bin_pt=4  float_type=Single  exp_bits=8  fraction_bits=24  en=off  latency=0  precision=User Defined  arith_type="Signed  (2's comp)"  n_bits=16  bin_pt=8  quantization=Truncate  overflow=Saturate  use_behavioral_HDL=off  mem_type=Block RAM  pipeline=off  XmcBlockStatus=1  maskContainerNames=tabcontainer1  block_type=cmult  block_config=sysgen:CMult_config
      settings: infoedit=[]
  CMult8 : hdlBasic/CMult  const=f(8)  gui_display_data_type=Fixed-point  const_n_bits=8  const_bin_pt=4  float_type=Single  exp_bits=8  fraction_bits=24  en=off  latency=0  precision=User Defined  arith_type="Signed  (2's comp)"  n_bits=16  bin_pt=8  quantization=Truncate  overflow=Saturate  use_behavioral_HDL=off  mem_type=Block RAM  pipeline=off  XmcBlockStatus=1  maskContainerNames=tabcontainer1  block_type=cmult  block_config=sysgen:CMult_config
      settings: infoedit=[]
  CMult9 : hdlBasic/CMult  const=f(7)  gui_display_data_type=Fixed-point  const_n_bits=8  const_bin_pt=4  float_type=Single  exp_bits=8  fraction_bits=24  en=off  latency=0  precision=User Defined  arith_type="Signed  (2's comp)"  n_bits=16  bin_pt=8  quantization=Truncate  overflow=Saturate  use_behavioral_HDL=off  mem_type=Block RAM  pipeline=off  XmcBlockStatus=1  maskContainerNames=tabcontainer1  block_type=cmult  block_config=sysgen:CMult_config
      settings: infoedit=[]
  Delay{1,7..13} (8 alike) : hdlBasic/Delay  rst=off  en=off  latency=1  reg_retiming=off  XmcBlockStatus=1  maskContainerNames=group1  block_type=delay  block_config=sysgen:Delay_config
  Transposed : hdlBasic/AddSub  mode=Addition  use_carryin=off  use_carryout=off  en=off  latency=0  precision=User Defined  arith_type="Signed  (2's comp)"  n_bits=16  bin_pt=8  quantization=Truncate  overflow=Saturate  use_behavioral_HDL=off  hw_selection=Fabric  pipelined=off  XmcBlockStatus=1  maskContainerNames=tabcontainer1  block_type=addsub  block_config=sysgen:Addsub_config
  Transposed1 : hdlBasic/AddSub  mode=Addition  use_carryin=off  use_carryout=off  en=off  latency=0  precision=User Defined  arith_type="Signed  (2's comp)"  n_bits=16  bin_pt=8  quantization=Truncate  overflow=Saturate  use_behavioral_HDL=off  hw_selection=Fabric  pipelined=off  XmcBlockStatus=1  maskContainerNames=tabcontainer1  block_type=addsub  block_config=sysgen:Addsub_config
  Out1 : Outport
  Out2 : Outport  Port=2
  wires:
  Delay12/1 -> AddSub12/2
  CMult10/1 -> AddSub9/1
  AddSub12/1 -> Delay13/1
  Delay9/1 -> AddSub9/2
  CMult9/1 -> AddSub7/1
  AddSub11/1 -> Delay12/1
  Delay10/1 -> AddSub10/2
  AddSub8/1 -> Delay9/1
  CMult11/1 -> AddSub8/1
  Delay8/1 -> AddSub8/2
  CMult12/1 -> AddSub10/1
  Delay11/1 -> AddSub11/2
  AddSub10/1 -> Delay11/1
  CMult14/1 -> AddSub12/1
  CMult15/1 -> Transposed/1
  Delay7/1 -> AddSub7/2
  CMult13/1 -> AddSub11/1
  Delay13/1 -> Transposed/2
  AddSub7/1 -> Delay8/1
  AddSub9/1 -> Delay10/1
  In1/1 -> CMult8/1, Out1/1, CMult15/1, CMult14/1, CMult13/1, CMult12/1, CMult10/1, CMult11/1, CMult9/1
  Transposed/1 -> Out2/1
  Transposed1/1 -> Delay7/1
  CMult8/1 -> Transposed1/1
  Delay1/1 -> Transposed1/2
  In2/1 -> Delay1/1
